simulink model "LACS"  (R2016b)
settings: Solver=VariableStepAuto  StartTime=0.0  StopTime=10  RelTol=1e-3
values from neighbouring files (symbols this model uses):
  coefficient = 0.8    [LACS.sldd]
  Detal_ref = 0.00022116955850615819 0.00022116955850615819 0.00024339323736781077 0.00026784369743330114 0.00029474273075037104 0.00032433393975435165 0.00035688482250496254 0.00039268904453642435 0.00043206891122917146 0.00047537805500027884 0.00052300435183202216 0.00057537308165349073 0.00063295034678974044 0.00069624676200566427 0.00076582142849131239 0.0008422862023284908 0.000926310265386283 0.0010186250    [LACS.sldd]    (also in path_generate.m = zeros(N,1))
  driver_decel = 4.0    [LACS.sldd]
  EgoLength = 3.048    [LACS.sldd]
  egopath = 0.0 0.25 0.5 0.75 1.0 1.25 1.5 1.7500000000000002 2.0 2.25 2.5 2.75 3.0 3.25 3.5000000000000004 3.75 4.0 4.25 4.5 4.75 5.0 5.25 5.5 5.75 6.0 6.25 6.5 6.75 7.0000000000000009 7.2499999999999991 7.5 7.75 8.0 8.25 8.5 8.75 9.0 9.25 9.5 9.75 10.0 10.25 10.5 10.75 11.0 11.25 11.5 11.75 12.0 12.25 12.5 12.75 13.0 13.25 13.5 13.750000000000002 14.000000000000002 14.250000000000002 14.499999999999998 14.7    [LACS.sldd]
  egoSpdLimit_H = 150.0    [LACS.sldd]
  egoSpdLimit_L = 10.0    [LACS.sldd]
  EgoWidth = 1.628    [LACS.sldd]
  ESA_Active = 3.0    [LACS.sldd]
  ESA_mask_1 = 31.0    [LACS.sldd]
  ESA_mask_2 = 15.0    [LACS.sldd]
  ESA_mask_3 = 255.0    [LACS.sldd]
  ESA_mask_4 = 31.0    [LACS.sldd]
  ESA_Passive = 1.0    [LACS.sldd]
  ESA_Standby = 2.0    [LACS.sldd]
  g = 9.8    [LACS.sldd]
  headwayoffset = 1.524    [LACS.sldd]
  LatAccelThershold = 0.05    [LACS.sldd]
  LatDis = 0.5    [LACS.sldd]
  LatSafetyThershold = 0.5    [LACS.sldd]
  LengthObj = 3.0    [LACS.sldd]
  ObjWidth = 2.0    [LACS.sldd]
  PB1_decel = 3.0    [LACS.sldd]
  PB2_decel = 5.0    [LACS.sldd]
  PB3_decel = 8.0    [LACS.sldd]
  Phi_dot_ref = 0.00085065224568106894 0.00085065224568106894 0.000936127966106986 0.0010301682404378703 0.0011336261186052523 0.0012474385378394444 0.001372634343205976 0.0015103430260158721 0.001661804233646022 0.0018283781058153412 0.0020115564932359636 0.0022129751145658549 0.0024344267064660809 0.0026778752189651235 0.0029454711038487576 0.0032395677369184911 0.0035627390050890382 0.0039177980756855638 0.004    [LACS.sldd]    (also in path_generate.m = zeros(N,1))
  Phi_ref = 0.00038406250525431664 0.00042271073336932769 0.00046524334565338114 0.00051204974395873044 0.000563558155980624 0.00062023946191088657 0.00068261138880285879 0.00075124310596315759 0.0008267602572639512 0.0009098504689462523 0.0010012693742370194 0.0011018471988988175 0.0012124959546271103 0.0013342172899504143 0.0014681110508986705 0.0016153846060911084 0.0017773629929370329 0.001955499943191484    [LACS.sldd]    (also in path_generate.m = phi_ref)
  SteerAngleLimit = 20.0    [LACS.sldd]
  SteerAngleSpdLimit = 20.0    [LACS.sldd]
  StrAngSpdThershold = 0.05    [LACS.sldd]
  StrAngThershold = 0.0    [LACS.sldd]
  Time2React = 1.2    [LACS.sldd]
  timeMargin = 0.5    [LACS.sldd]
  TTCthreshold1 = 2.5    [LACS.sldd]
  TTCthreshold3 = 1.0    [LACS.sldd]
  X_dot_ref = 10.0 10.0 10.0 9.9999999999999947 10.0 10.0 10.0 10.0 10.0 10.0 10.0 10.0 10.0 10.0 10.0 10.000000000000018 10.0 10.0 10.0 10.0 10.0 10.0 10.0 10.0 10.0 10.0 10.0 10.0 10.0 10.0 10.0 10.0 10.0 10.0 10.0 10.0 10.0 10.0 10.0 10.0 10.0 10.0 10.0 10.0 10.0 10.0 10.0 10.0 10.0 10.0 10.0 10.0 10.0 10.0 10.0 10.0 10.0 10.0 10.0 10.0 10.0 10.0 10.0 9.9999999999999289 10.0 10.0 10.0 10.0 10.0 10.0 10.0 10.    [LACS.sldd]    (also in path_generate.m = zeros(N,1))
  X_ref = 0.05 0.55 1.05 1.55 2.05 2.55 3.05 3.55 4.05 4.55 5.05 5.55 6.05 6.55 7.05 7.55 8.05 8.55 9.05 9.55 10.05 10.55 11.05 11.55 12.05 12.55 13.05 13.55 14.05 14.55 15.05 15.55 16.05 16.55 17.05 17.55 18.05 18.55 19.05 19.55 20.05 20.55 21.05 21.55 22.05 22.55 23.05 23.55 24.05 24.55 25.05 25.55 26.05 26.55 27.05 27.55 28.05 28.55 29.05 29.55 30.05 30.55 31.05 31.55 32.05 32.55 33.05 33.55 34.05 34.55    [LACS.sldd]    (also in path_generate.m = X_phi')
  Y_dot_ref = 0.0044363771042237217 0.0044363771042237217 0.00488273213335339 0.0053739322979981 0.0059144698111347933 0.0065092840662692251 0.0071638055584438178 0.0078840039934084845 0.0086764409570179273 0.0095483275445279979 0.01050758737719603 0.011562925461771293 0.012723903376023141 0.014001021290828194 0.015405807364013962 0.016950915064438028 0.018650229002128878 0.020518979854070446 0.0225738689793052    [LACS.sldd]    (also in path_generate.m = zeros(N,1))
  Y_ref = 0.0020016327462461514 0.0022031718511841521 0.0024249907063953382 0.0026691273130630077 0.0029378239279629127 0.0032335474185196523 0.0035590116218331136 0.0039172018997553045 0.0043114020994257287 0.0047452241472766251 0.005222640524503025 0.0057480198933628265 0.0063261661664513911 0.0069623613352525482 0.0076624123997939579 0.008432702767994656 0.0092802485212165574 0.010212759971323001 0.01123    [LACS.sldd]    (also in path_generate.m = zeros(N,1))
undefined symbols (not defined in the file or in its folder): ADR_ADRCycleTime, ADR_SteeringYawrateThresh_p, AEB_mask1, aubr, CAEB_AccelPdlPosLimit, CAEB_AccelPdlPosSpdThreshold, CAEB_CalAEBLongVelObjLimit_mps, CAEB_CalAEBVMaxDec_kmph, ESA_AESACTIVE, ESA_ERROR, ESA_ESAFunctionOFF, ESA_ESAFunctionON, ESA_ESASwichOFF, ESA_ESS_DriverSteeringNumThreshold, ESA_ESSACTIVE, ESA_ForewardCollissionLevel2, ESA_ForewardCollissionLevel3, ESA_OFF, ESA_PASSIVE, ESA_PLAN_AES, ESA_PLAN_ESSLEFT, ESA_PLAN_ESSRIGHT, ESA_PLAN_FAILURE, ESA_PLAN_OFF, ESA_PLAN_STANDBY, ESA_PLAN_WAIT, ESA_SPEEDLIMITH6_p, ESA_SPEEDLIMITH7_p, ESA_SPEEDLIMITL6_p, ESA_SPEEDLIMITL7_p, ESA_STANDBY, ESA_StrAngSpdT6_p, FromAngle2Rad, Kp, magnitude, tablebr, TTCthreshold, vubr
libraries: simulink x15, Solver_SF x9, simulink_extras x1
(part 1 of 5)
settings Model: DataDictionary=LACS.sldd  NumberOfSteps=100  Creator=NEUSOFT  LastModifiedBy=NEUSOFT

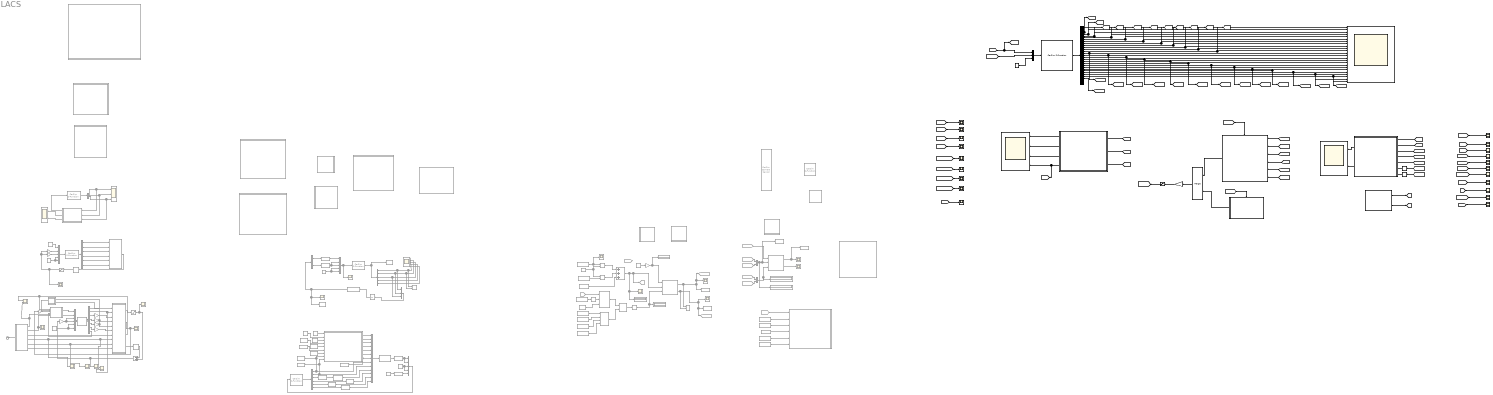
== system LACS ==
  note: 输入是制动压力
  note: 规划接口
  note: 转向不足
  note: 判断条件：
      | 1.前车静止或运动，自车与前车的关系
      | 2.TTC
      | 3.目标纵向速度
      | 4.目标纵向距离
      | 5.自车速度
      | 6.方向盘角度
      | 7.方向盘角速度
      | 8.没有刹车动作
      | 9.没有急加速动作
      | 10.航向角判断
  AEB : Subsystem  Commented=on
  AEB/ESA Comprehensive Decision : Stateflow chart  Commented=on  TreatAsAtomicUnit=on
  AEB/ESA Comprehensive Decision1 : Stateflow chart  Commented=on  TreatAsAtomicUnit=on
  AEB/ESAModeSwitch : Subsystem  Commented=on
  AEB_System : Subsystem  Commented=on
  AEBsts : Subsystem
  Add : Sum  Commented=on  Inputs=-+
  Add1 : Sum  Commented=on  Inputs=+++
  Bus Creator : BusCreator  Commented=on  Inputs=2
  Bus Creator1 : BusCreator  Commented=on  Inputs=2
  CTRL : Subsystem  Commented=on
  CarSim Camera Sensor : Solver_SF/CarSim Camera Sensor  Priority=1  Commented=on
  CarSim S-Function : Solver_SF/CarSim S-Function  Priority=1  Commented=on  SIMFILE=Simfile.sim
  CarSim S-Function1 : Solver_SF/CarSim S-Function  Priority=1  Commented=on  SIMFILE=simfile.sim
  CarSim S-Function2 : Solver_SF/CarSim S-Function  Priority=1  Commented=on  SIMFILE=simfile.sim
  CarSim S-Function2v : Solver_SF/CarSim S-Function2v  Priority=1  Commented=on  SIMFILE=[]
  CarSim S-Function3 : Solver_SF/CarSim S-Function  Priority=1  SIMFILE=simfile.sim
  CarSim S-Function4 : Solver_SF/CarSim S-Function  Priority=1  Commented=on  SIMFILE=simfile
  CarSim S-Function5 : Solver_SF/CarSim S-Function  Priority=1  Commented=on  SIMFILE=simfile.sim
  CarSim S-Function6 : Solver_SF/CarSim S-Function  Priority=1  Commented=on  SIMFILE=[]
  Clock : Clock  Commented=on
  Constant{,2,4,28} (4 alike) : Constant  Commented=on  Value=0
  Constant1 : Constant  Commented=on  Value=0.15
  Constant10 : Constant  Commented=on  Value=0.67
  Constant11 : Constant  Commented=on  Value=3
  Constant12 : Constant  Commented=on  Value=3
  Constant13 : Constant  Commented=on  Value=10
  Constant14 : Constant  Commented=on  Value=ObjWidth
  Constant15 : Constant  Commented=on  Value=10
  Constant16 : Constant  Commented=on  Value=EgoWidth
  Constant17 : Constant  Commented=on  Value=LatDis
  Constant18 : Constant  Commented=on  Value=coefficient
  Constant19 : Constant  Commented=on  Value=g
  Constant20 : Constant  Commented=on  Value=ObjWidth
  Constant21 : Constant  Commented=on  Value=X_ref
  Constant22 : Constant  Commented=on  Value=Y_ref
  Constant23 : Constant  Commented=on  Value=Phi_ref
  Constant24 : Constant  Commented=on  Value=X_dot_ref
  Constant25 : Constant  Commented=on  Value=Y_dot_ref
  Constant26 : Constant  Commented=on  Value=Phi_dot_ref
  Constant27 : Constant  Commented=on  Value=Detal_ref
  Constant29 : Constant  Commented=on  Value=10
  Constant30 : Constant  Value=0.5
  Constant5 : Constant  Commented=on  Value=1.5
  Constant6 : Constant  Commented=on  Value=0.5
  Constant7 : Constant  Commented=on  Value=2
  Constant8 : Constant  Commented=on  Value=0.8
  Constant9 : Constant  Commented=on  Value=9.8
  Delay : Delay  Commented=on  DelayLength=1  UseCircularBuffer=on
  Delay1 : Delay  DelayLength=1
  Delay2 : Delay  DelayLength=1
  Demux : Demux  Commented=on  Outputs=3
  Demux1 : Demux  Commented=on  Outputs=6
  Demux2 : Demux  Commented=on  Outputs=7
  Demux3 : Demux  Outputs=25
  Demux4 : Demux  Commented=on  Outputs=2
  Demux5 : Demux  Commented=on  Outputs=5
  Demux6 : Demux  Commented=on  Outputs=6
  Display{,1..4} (5 alike) : Display  Commented=on
  Divide : Product  Commented=on  Inputs=*/
  Divide1 : Product  Commented=on  Inputs=/*
  Divide2 : Product  Commented=on  Inputs=****
  Divide3 : Product  Commented=on  Inputs=***
  Divide4 : Product  Commented=on  Inputs=*/
  ESA : Subsystem  Commented=on
  ESAManager : Stateflow chart  Commented=on  TreatAsAtomicUnit=on
  ESARegulator_NOTON : Subsystem
  ESARegurator_ON : Subsystem
  ESAsts : Subsystem
  Fcn : Fcn  Commented=on  Expr=u*3.6
  Fcn1 : Fcn  Commented=on  Expr=u*180/pi
  Fcn2 : Fcn  Commented=on  Expr=u/180*pi
  Fcn3 : Fcn  Commented=on  Expr=u/pi*180
  Fcn4 : Fcn  Commented=on  Expr=u*3.6
  Fcn5 : Fcn  Commented=on  Expr=u/3.6
  Fcn6 : Fcn  Commented=on  Expr=u/3.6
  Fcn7 : Fcn  Commented=on  Expr=u/180*pi
  From17 : From  Commented=on  GotoTag=ye  TagVisibility=global
  From18 : From  Commented=on  GotoTag=egoSpd  TagVisibility=global
  From19 : From  Commented=on  GotoTag=egoSpd  TagVisibility=global
  From20 : From  Commented=on  GotoTag=L_prepoint  TagVisibility=global
  From21 : From  Commented=on  GotoTag=Xo  TagVisibility=global
  From22 : From  Commented=on  GotoTag=Yo  TagVisibility=global
  From23 : From  Commented=on  GotoTag=ego_path_x
  From24 : From  Commented=on  GotoTag=ego_path_y
  Gain : Gain  Commented=on  Gain=180/pi
  Gain1 : Gain  Commented=on  Gain=180/pi
  Gain2 : Gain  Commented=on  Gain=1/3.6
  Gain3 : Gain  Commented=on  Gain=1/3.6
  Gain4 : Gain  Commented=on  Gain=pi/180
  Gain5 : Gain  Commented=on  Gain=180/pi
  Gain6 : Gain  Commented=on  Gain=pi/180
  Gain7 : Gain  Commented=on  Gain=-1
  Gain8 : Gain  Gain=15.6
  Gain9 : Gain  Commented=on  Gain=1/3.6
  Goto26 : Goto  Commented=on  GotoTag=ye  TagVisibility=global
  Goto27 : Goto  Commented=on  GotoTag=ego_path_x
  Goto28 : Goto  Commented=on  GotoTag=ego_path_y
  LQR : Subsystem  Commented=on
  LatParamCaculation : Subsystem
  MATLAB Function : MATLAB Function  Commented=on  TreatAsAtomicUnit=on
  MATLAB Function1 : MATLAB Function  Commented=on  TreatAsAtomicUnit=on
  MATLAB Function2 : MATLAB Function  Commented=on  TreatAsAtomicUnit=on
  Merge : Merge
  Mux : Mux  Commented=on  Inputs=5
  Mux1 : Mux  Commented=on  Inputs=6
  Mux2 : Mux  Inputs=3
  Mux3 : Mux  Commented=on  Inputs=5
  Mux4 : Mux  Commented=on  Inputs=3
  Mux5 : Mux  Commented=on  Inputs=13
  Mux6 : Mux  Commented=on  Inputs=5
  PID Controller : simulink/Continuous/PID Controller  Commented=on  Controller=PID  TimeDomain=Continuous-time  SampleTime=-1  IntegratorMethod=Forward Euler  FilterMethod=Forward Euler  Form=Parallel  UseFilter=on  ControllerParametersSource=internal  P=0  I=0  D=0  N=100  InitialConditionSource=internal  InitialConditionForIntegrator=0  InitialConditionForFilter=0  ExternalReset=none  LimitOutput=off  UpperSaturationLimit=inf  LowerSaturationLimit=-inf  LinearizeAsGain=on  AntiWindupMode=none  Kb=1  TrackingMode=off  Kt=1  PParamMin=[]  PParamMax=[]  IParamMin=[]  IParamMax=[]  DParamMin=[]  DParamMax=[]  NParamMin=[]  NParamMax=[]  KbParamMin=[]  KbParamMax=[]  KtParamMin=[]  KtParamMax=[]  POutMin=[]  POutMax=[]  IOutMin=[]  IOutMax=[]  DOutMin=[]  DOutMax=[]  NOutMin=[]  NOutMax=[]  KbOutMin=[]  KbOutMax=[]  KtOutMin=[]  KtOutMax=[]  IntegratorOutMin=[]  IntegratorOutMax=[]  FilterOutMin=[]  FilterOutMax=[]  SumOutMin=[]  SumOutMax=[]  SumI1OutMin=[]  SumI1OutMax=[]  SumI2OutMin=[]  SumI2OutMax=[]  SumI3OutMin=[]  SumI3OutMax=[]  SumDOutMin=[]  SumDOutMax=[]  SaturationOutMin=[]  SaturationOutMax=[]  IntegratorContinuousStateAttributes=''  IntegratorStateMustResolveToSignalObject=off  IntegratorRTWStateStorageClass=Auto  FilterContinuousStateAttributes=''  FilterStateMustResolveToSignalObject=off  FilterRTWStateStorageClass=Auto  DifferentiatorICPrevScaledInput=0  DifferentiatorOutMin=[]  DifferentiatorOutMax=[]
  PassengerAEBManagement : Stateflow chart  Commented=on  TreatAsAtomicUnit=on
  Planning&Controlling : Subsystem  Commented=on
  S-Function : S-Function  Commented=on  FunctionName=MPC_Controller  SFunctionDeploymentMode=off  EnableBusSupport=off
  S-Function1 : S-Function  Commented=on  FunctionName=mpc_controller  SFunctionDeploymentMode=off  EnableBusSupport=off
  Saturation : Saturate  Commented=on  UpperLimit=1.2  LowerLimit=-1.2
  Saturation1 : Saturate  Commented=on  UpperLimit=1  LowerLimit=-1
  Saturation2 : Saturate  UpperLimit=180  LowerLimit=-180
  Scope : Scope  Commented=on  NumInputPorts=3
  Scope1 : Scope  Commented=on  NumInputPorts=2
  Scope{2,4..6,8..10,14,16..20,29..30} (15 alike) : Scope  Commented=on
  Scope11 : Scope  NumInputPorts=24
  Scope12 : Scope  NumInputPorts=4
  Scope13 : Scope  NumInputPorts=2
  Scope15 : Scope  Commented=on  NumInputPorts=5
  Scope{21..28,31..42} (20 alike) : Scope
  Scope3 : Scope  Commented=on  NumInputPorts=2
  Scope7 : Scope  Commented=on  NumInputPorts=2
  Sqrt : Sqrt  Commented=on  SaturateOnIntegerOverflow=on
  Sqrt1 : Sqrt  Commented=on  SaturateOnIntegerOverflow=on
  Subsystem : Subsystem  Commented=on
  To Workspace : ToWorkspace  Commented=on  VariableName=u  SaveFormat=Timeseries  SampleTime=-1
  To Workspace1 : ToWorkspace  Commented=on  VariableName=y  SaveFormat=Timeseries  SampleTime=-1
  To Workspace2 : ToWorkspace  Commented=on  VariableName=ego_path_y  SaveFormat=Structure With Time  SampleTime=-1
  To Workspace3 : ToWorkspace  Commented=on  VariableName=simout1  SaveFormat=Structure With Time  SampleTime=-1
  To Workspace4 : ToWorkspace  Commented=on  VariableName=ego_path_x  SaveFormat=Structure With Time  SampleTime=-1
  To Workspace5 : ToWorkspace  Commented=on  VariableName=simout2  SaveFormat=Structure With Time  SampleTime=-1
  To Workspace6 : ToWorkspace  Commented=on  VariableName=car_x  SampleTime=0.1
      settings: Save2DSignal=2-D array (concatenate along first dimension)
  To Workspace7 : ToWorkspace  Commented=on  VariableName=car_y  SampleTime=0.1
      settings: Save2DSignal=2-D array (concatenate along first dimension)
  To Workspace8 : ToWorkspace  Commented=on  VariableName=car_steer  SampleTime=0.1
      settings: Save2DSignal=2-D array (concatenate along first dimension)
  TroqueOutput : Subsystem  Commented=on
  Unit Delay : UnitDelay  Commented=on  SampleTime=-1
  XY Graph : simulink/Sinks/XY Graph  Commented=on  xmin=-1  xmax=1  ymin=-1  ymax=1  st=-1
  XY Graph1 : simulink/Sinks/XY Graph  Commented=on  xmin=-10  xmax=10  ymin=-10  ymax=10  st=-1
  double_pid_controller : Subsystem  Commented=on
  planning : MATLAB Function  Commented=on  TreatAsAtomicUnit=on
  trajectoryPlanning1 : MATLAB Function  Commented=on  TreatAsAtomicUnit=on
  trajectoryPlanning2 : MATLAB Function  Commented=on  TreatAsAtomicUnit=on
  trajectoryPlanning3 : MATLAB Function  Commented=on  TreatAsAtomicUnit=on
  trajectoryPlanning4 : MATLAB Function  Commented=on  TreatAsAtomicUnit=on
  trajectoryPlanning5 : MATLAB Function  Commented=on  TreatAsAtomicUnit=on
  trajectoryPlanning6 : MATLAB Function  Commented=on  TreatAsAtomicUnit=on
  tag scope: Angle_C2C=global, Angle_C2L=global, Angle_C2R=global, Angle_ego2obj=global, Dis_rel=global, ID_Obj=global, L_prepoint=global, L_x=global, LatAcc=global, LongiAcc=global, Mng_Obj=global, Spd_rel=global, SteerAngSpd=global, SteerAngle=global, Warning_L=global, Warning_R=global, Width_Obj=global, Xo=global, Xo_Obj=global, Yaw=global, YawRate=global, Yo=global, Yo_Obj=global, egoSpd=global, egospd_y=global
  wires:
  AEB_System/1(CMpa) -> CarSim S-Function/1
  CarSim S-Function/1 -> Demux/1
  Demux/1 -> AEB_System/1(Distance), Scope/1
  Demux/2 -> Scope/2, AEB_System/2(V_difference)
  Demux/3 -> AEB_System/3("V_Speed "), Scope/3
  AEB_System/2("Alart ") -> Scope1/1
  AEB_System/3("Break_signal ") -> Scope1/2
  CarSim S-Function1/1 -> Demux1/1
  Mux/1 -> CarSim S-Function1/1
  Demux1/1 -> Subsystem/1(x)  "x"
  Demux1/2 -> Subsystem/2(y)  "y"
  Demux1/3 -> Subsystem/3(phi)  "phi"
  Demux1/4 -> Subsystem/4(vx)  "vx"
  Demux1/5 -> Subsystem/5(vy)  "vy"
  Demux1/6 -> Subsystem/6(phi_dot)  "phi_dot"
  Subsystem/1(angle) -> Delay/1
  Gain/1 -> Mux/2
  Gain1/1 -> Mux/3
  Delay/1 -> Saturation/1
  Constant/1 -> Mux/4, Mux/5
  Constant1/1 -> Mux/1
  Saturation/1 -> Scope2/1, Gain1/1, Gain/1
  CarSim S-Function2/1 -> Demux2/1
  Mux1/1 -> CarSim S-Function2/1
  Demux2/1 -> LQR/1(x)  "x"
  Demux2/2 -> Scope3/2, LQR/2(y)  "y"
  Demux2/3 -> Gain4/1  "yaw"
  Demux2/4 -> Gain2/1  "vx"
  Demux2/5 -> Gain3/1  "vy"
  Demux2/6 -> Gain6/1  "dyaw"
  Gain3/1 -> MATLAB Function/2(vy), LQR/5(vy)
  Gain4/1 -> LQR/3(phi)
  Gain6/1 -> LQR/6(phi_dot)
  Demux2/7 -> double_pid_controller/4(rpm)  "rpm"
  double_pid_controller/1(Out1) -> Mux1/1
  double_pid_controller/2(Out2) -> Mux1/2
  Gain2/1 -> MATLAB Function/1(vx), LQR/4(vx)
  MATLAB Function/1(v) -> double_pid_controller/2(v)
  Clock/1 -> planning/1(t)
  planning/1(vp) -> Scope7/2, double_pid_controller/5(vp)  "vp"
  planning/2(ap) -> Scope6/1, double_pid_controller/6(ap)  "ap"
  planning/3(xr) -> LQR/7(xr)
  planning/4(yr) -> Scope8/1, Scope3/1, LQR/8(yr)
  planning/5(thetar) -> Scope9/1, LQR/9(thetar)
  LQR/3(s_dot) -> double_pid_controller/1(s_dot), Scope7/1
  LQR/2(es) -> Scope5/1, Gain7/1
  LQR/1(angle) -> Saturation1/1
  Constant2/1 -> Mux1/5, Mux1/6
  Gain7/1 -> double_pid_controller/3(es)
  LQR/4(ed) -> PID Controller/1
  PID Controller/1 -> Add/1
  Saturation1/1 -> Scope4/1, Add/2
  Add/1 -> Scope10/1, Gain5/1
  Gain5/1 -> Mux1/4, Mux1/3
  planning/6(kr) -> LQR/10(kappar)
  Mux2/1 -> CarSim S-Function3/1
  AEBsts/4(decel) -> [CMpa], Scope12/4
  AEBsts/3(AEBsts) -> Scope12/3
  AEBsts/2(FCW_Active) -> Scope12/2
  AEBsts/1(collision) -> Scope12/1
  CarSim S-Function3/1 -> Demux3/1
  Demux3/23 -> [Yo_Obj], Scope11/23  "目标物的横坐标"
  Demux3/22 -> [Xo_Obj], Scope11/22  "目标物的纵坐标"
  Demux3/20 -> [L_prepoint], Scope11/20  "纵向预瞄点"
  Demux3/24 -> [SteerAngSpd], Scope11/24  "方向盘角速度"
  Demux3/21 -> [L_x], Scope11/21  "纵坐标"
  Demux3/19 -> [Yo], Scope11/19  "车辆质心的全局Y坐标"
  Demux3/18 -> [Xo], Scope11/18  "车辆质心的全局X坐标"
  Demux3/17 -> [YawRate], Scope11/17  "车辆航向角的导数"
  Demux3/16 -> [LatAcc], Scope11/16  "横向加速度"
  Demux3/15 -> [LongiAcc], Scope11/15  "纵向加速度"
  Demux3/14 -> [Yaw], Scope11/14  "航向角"
  Demux3/13 -> [SteerAngle], Scope11/13  "方向盘转角"
  Demux3/12 -> [Angle_ego2obj], Scope11/12  "本车与物体垂向的方位角"
  Demux3/11 -> [Angle_C2R], Scope11/11  "相对传感器瞄准的方向，到物体最右侧直线的方位角"
  Demux3/10 -> [Angle_C2L], Scope11/10  "相对传感器瞄准的方向，到物体最左侧直线的方位角"
  Demux3/9 -> [Angle_C2C], Scope11/9  "相对传感器瞄准的方向，到物体最近点直线的方位角"
  Demux3/8 -> [Warning_R], Scope11/8  "右侧预警"
  Demux3/7 -> [Warning_L], Scope11/7  "左侧预警"
  Demux3/6 -> [Mng_Obj], Scope11/6  "置信度"
  Demux3/5 -> [Width_Obj], Scope11/5  "目标宽度"
  Demux3/4 -> [ID_Obj], Scope11/4  "目标ID"
  Demux3/3 -> Scope11/3, [egoSpd]  "纵向速度"
  Demux3/2 -> Scope11/2, [Spd_rel]  "相对速度"
  Demux3/1 -> [Dis_rel], Scope11/1  "相对距离"
  [ESA_Active] -> ESARegurator_ON/Action
  [ESA_NOTActive] -> ESARegulator_NOTON/Action
  ESARegurator_ON/1(WheelSteerAngle) -> Merge/1
  ESARegulator_NOTON/1(WheelSteerAngle) -> Merge/2
  ESAsts/2(ESAsts) -> Scope13/2
  Merge/1 -> Gain8/1
  [Dis_rel] -> AEBsts/1(LongiDis)
  [Spd_rel] -> AEBsts/2(LongiVel)
  [egoSpd] -> AEBsts/3(EgoSpd)
  [Dis_rel] -> ESAsts/1(LongiDis)
  [Spd_rel] -> ESAsts/2(LongiVel)
  [SteerAngSpd] -> ESAsts/4(SteerAngleSpd)
  [SteerAngle] -> ESAsts/3(SteerAngle)
  [LatAcc] -> ESAsts/5(LatAccel)
  Mux3/1 -> Scope16/1, CarSim S-Function4/1
  Fcn/1 -> Mux3/1  "Speed"
  Fcn1/1 -> Mux3/3, Mux3/2  "Steer_R1"
  Constant4/1 -> Mux3/5, Mux3/4  "Steer_R2"
  Demux4/1 -> Fcn/1  "V"
  Demux4/2 -> Fcn1/1  "δ"
  S-Function/1 -> Scope14/1, To Workspace/1, Demux4/1
  Unit Delay/1 -> S-Function/1
  CarSim S-Function4/1 -> Demux5/1, To Workspace1/1
  Demux5/1 -> Mux4/1, XY Graph/1, Scope15/1  "X0"
  Demux5/2 -> Mux4/2, XY Graph/2, Scope15/2  "Y0"
  Demux5/3 -> Mux4/3, Scope15/3  "Yaw"
  Demux5/4 -> Scope15/4  "Vx"
  Demux5/5 -> Scope15/5  "Steer_SW"
  Mux4/1 -> Unit Delay/1
  [CMpa] -> [CMpa_M], Mux2/1
  [SteerAngle_Out] -> Mux2/2
  Constant14/1 -> Scope29/1, Divide/1
  Constant7/1 -> Divide/2, Divide1/1
  Constant5/1 -> Divide1/2
  Divide1/1 -> Add1/2
  Divide/1 -> Add1/1
  Constant6/1 -> Add1/3
  Add1/1 -> Display4/1, Scope30/1, trajectoryPlanning2/2(ye), Goto26/1
  Constant11/1 -> Divide2/4
  Constant10/1 -> Divide2/3
  Constant9/1 -> Divide2/2
  Constant8/1 -> Divide2/1
  From17/1 -> Divide3/1
  Sqrt/1 -> Divide3/2
  Constant12/1 -> Sqrt/1
  Constant13/1 -> Divide3/3
  Divide3/1 -> Divide4/1
  Divide2/1 -> Divide4/2
  Divide4/1 -> Sqrt1/1
  Sqrt1/1 -> trajectoryPlanning2/3(te), Display/1
  Gain9/1 -> trajectoryPlanning2/1(v_x), Display1/1
  trajectoryPlanning2/1(egopath_x) -> XY Graph1/1, Goto27/1, Scope18/1, To Workspace4/1
  trajectoryPlanning2/2(egopath_y) -> XY Graph1/2, Scope17/1, Goto28/1, To Workspace2/1
  From20/1 -> trajectoryPlanning3/1(ld_veh)
  From21/1 -> Bus Creator/1
  From22/1 -> Bus Creator/2
  Bus Creator/1 -> Display2/1, trajectoryPlanning3/3("currentPose ")
  From23/1 -> Bus Creator1/1
  From24/1 -> Bus Creator1/2
  trajectoryPlanning3/1(ld_pre) -> To Workspace5/1, Scope19/1
  Bus Creator1/1 -> Display3/1, trajectoryPlanning3/2(refpath), To Workspace3/1
  trajectoryPlanning3/2(currentPose) -> Scope20/1
  [te] -> Delay2/1
  [ye] -> Delay1/1
  Delay2/1 -> ESAsts/7(te)
  [TTC_M] -> Scope23/1
  [CMpa_M] -> Scope21/1
  [Longivel_M] -> Scope24/1
  [LongiDis_M] -> Scope25/1
  [FCWStopTime_M] -> Scope22/1
  [PB1StoppingTime_M] -> Scope26/1
  [PB2StoppingTime_M] -> Scope27/1
  [FBStoppingTime] -> Scope28/1
  [ESA_sts_M] -> Scope31/1
  [Dis_rel] -> Scope32/1
  [Spd_rel] -> Scope33/1
  [SteerAngle] -> Scope34/1
  [SteerAngle_Out] -> Scope37/1
  [LatAcc] -> Scope36/1
  [SteerAngSpd] -> Scope35/1
  [LatDisLimit_c] -> Scope40/1
  [TTC] -> Scope39/1
  [Allow2Str] -> Scope38/1
  ESAsts/1(collision) -> Scope13/1
  Delay1/1 -> ESAsts/6(ye)
  Gain8/1 -> Saturation2/1
  Saturation2/1 -> [SteerAngle_Out]
  Constant15/1 -> Gain9/1
  Constant19/1 -> trajectoryPlanning6/6(g)
  Constant18/1 -> trajectoryPlanning6/5(coefficient)
  Constant17/1 -> trajectoryPlanning6/4(EgoWidth)
  Constant16/1 -> trajectoryPlanning6/3(ObjWidth)
  Constant20/1 -> trajectoryPlanning6/2(LatDis)
  From18/1 -> trajectoryPlanning6/1(v_x)
  Constant21/1 -> MATLAB Function1/1(X_ref)
  Constant22/1 -> MATLAB Function1/2(Y_ref)
  Constant23/1 -> MATLAB Function1/3(Phi_ref)
  Constant24/1 -> MATLAB Function1/4(X_dot_ref)
  Constant25/1 -> MATLAB Function1/5(Y_dot_ref)
  Constant26/1 -> MATLAB Function1/6(Phi_dot_ref)
  Constant27/1 -> MATLAB Function1/7(Detal_ref)
  MATLAB Function1/5(y_dot_ref) -> Mux5/5
  MATLAB Function1/1(x_ref) -> Mux5/1
  MATLAB Function1/2(y_ref) -> Mux5/2
  MATLAB Function1/3(phi_ref) -> Mux5/3
  MATLAB Function1/4(x_dot_ref) -> Mux5/4
  MATLAB Function1/6(phi_dot_ref) -> Mux5/6
  MATLAB Function1/7(detal_ref) -> To Workspace8/1, Mux5/7
  Mux5/1 -> S-Function1/1
  CarSim S-Function5/1 -> Demux6/1
  Demux6/1 -> MATLAB Function1/8(x), To Workspace6/1, Mux5/8
  Demux6/2 -> MATLAB Function1/9(y), To Workspace7/1, Mux5/9
  Demux6/4 -> Fcn5/1
  Demux6/5 -> Fcn6/1
  Demux6/6 -> Fcn7/1
  Demux6/3 -> Fcn2/1
  Fcn2/1 -> MATLAB Function2/1(u)
  MATLAB Function2/1(yaw) -> Mux5/10
  Constant28/1 -> Mux6/3, Mux6/4
  Fcn3/1 -> Mux6/1, Mux6/2
  S-Function1/1 -> Fcn3/1
  Constant29/1 -> Fcn4/1
  Fcn4/1 -> Mux6/5
  Mux6/1 -> CarSim S-Function5/1
  Fcn5/1 -> Mux5/11
  Fcn6/1 -> Mux5/12
  Fcn7/1 -> Mux5/13
  Constant30/1 -> Mux2/3
  LatParamCaculation/2(te) -> [te]
  LatParamCaculation/1(ye) -> [ye]
  [Xo] -> ESARegurator_ON/1(Xo)
  [Yo] -> ESARegurator_ON/2(Yo)
  [Yaw] -> ESARegurator_ON/3(Yaw)
  [YawRate] -> ESARegurator_ON/6(YawRate)
  Demux3/25 -> [egospd_y]
  [egoSpd] -> ESARegurator_ON/4(X_dot)
  [egospd_y] -> ESARegurator_ON/5(Y_dot)
  [egoSpd] -> Scope41/1
  [egoSpd] -> Scope42/1

== system LACS/AEB ==
  LongiVel : Inport
  LongiDis : Inport  Port=2
  ConditionAdaptAEB : Subsystem
  DrvRapidAccelAction : Subsystem  Commented=on
  TTCCaculation : Subsystem
  Out1 : Outport
  Out3 : Outport  Port=2
  Out4 : Outport  Port=3
  Out5 : Outport  Port=4
  Out6 : Outport  Port=5
  Out7 : Outport  Port=6
  Out8 : Outport  Port=7
  Out10 : Outport  Port=8
  wires:
  ConditionAdaptAEB/6(Out6) -> Out7/1
  ConditionAdaptAEB/5(Out5) -> Out6/1
  ConditionAdaptAEB/2(Out2) -> Out3/1
  ConditionAdaptAEB/8(Out8) -> Out10/1
  ConditionAdaptAEB/7(Out7) -> Out8/1
  ConditionAdaptAEB/3(Out3) -> Out4/1
  ConditionAdaptAEB/1(Out1) -> Out1/1
  ConditionAdaptAEB/4(Out4) -> Out5/1
  LongiVel/1 -> TTCCaculation/1(LongiVel)
  LongiDis/1 -> TTCCaculation/2(LongiDis)

== system LACS/AEB//ESAModeSwitch ==
  SteerAngle : Inport
  SteerAngleSpd : Inport  Port=2
  AEBTTC : Inport  Port=3
  EgoSpd : Inport  Port=4
  If : If  IfExpression=u1==1
  If Action Subsystem : Subsystem  TreatAsAtomicUnit=on
  If Action Subsystem1 : Subsystem  TreatAsAtomicUnit=on
  Merge : Merge
  Merge1 : Merge
  Relational Operator22 : RelationalOperator  Operator=<=  OutDataTypeStr=boolean  RndMeth=Simplest
  Subsystem : Subsystem
  TTC1 : Constant  Value=6  OutDataTypeStr=boolean
  ESATakeOverReq : Outport
  AEBCrashAvoid : Outport  Port=2
  wires:
  If/1 -> If Action Subsystem/Action
  If/2 -> If Action Subsystem1/Action
  SteerAngle/1 -> Subsystem/1(SteerAngle)
  SteerAngleSpd/1 -> Subsystem/2(SteerAngleSpd)
  Subsystem/1(DrvRapidSteerAction) -> If/1
  EgoSpd/1 -> If Action Subsystem1/2(EgoSpd)
  AEBTTC/1 -> If Action Subsystem1/3(AEBTTC), Relational Operator22/1
  TTC1/1 -> Relational Operator22/2
  Relational Operator22/1 -> If Action Subsystem1/1(AEBTTCVaild)
  Merge/1 -> ESATakeOverReq/1
  Merge1/1 -> AEBCrashAvoid/1
  If Action Subsystem/1(ESAVTakeOverReq) -> Merge/1
  If Action Subsystem1/1(ESAVTakeOverReq) -> Merge/2
  If Action Subsystem/2(AEBVCrashAvoid) -> Merge1/1
  If Action Subsystem1/2(AEBVCrashAvoid) -> Merge1/2

== system LACS/AEB_System ==
  Distance : Inport
  V_difference : Inport  Port=2
  "V_Speed " : Inport  Port=3
  Chart : Stateflow chart  TreatAsAtomicUnit=on
  CMpa : Outport
  "Alart " : Outport  Port=2
  "Break_signal " : Outport  Port=3
  wires:
  Distance/1 -> Chart/1(Distance)
  V_difference/1 -> Chart/2(V_difference)
  "V_Speed "/1 -> Chart/3(V_Speed)
  Chart/1(CMpa) -> CMpa/1
  Chart/2(Alart) -> "Alart "/1
  Chart/3(Break_signal) -> "Break_signal "/1

== system LACS/AEBsts ==
  LongiDis : Inport
  LongiVel : Inport  Port=2
  EgoSpd : Inport  Port=3
  AEB_sts : Stateflow chart  TreatAsAtomicUnit=on
  Brake2StopTime : Subsystem
  Constant1 : Constant  Value=PB2_decel
  Constant2 : Constant  Value=PB3_decel
  Constant3 : Constant  Value=PB1_decel
  Constant6 : Constant  Value=0.1
  Relational Operator4 : RelationalOperator  Operator=<  OutDataTypeStr=boolean  RndMeth=Simplest
  TTCCaculation : Subsystem
  collision : Outport
  FCW_Active : Outport  Port=2
  AEBsts : Outport  Port=3
  decel : Outport  Port=4
  wires:
  TTCCaculation/1(collision) -> collision/1
  EgoSpd/1 -> Relational Operator4/1, Brake2StopTime/1(EgoSpd)
  Constant3/1 -> AEB_sts/6(CMpa1), Brake2StopTime/2(CMpa1)
  Constant1/1 -> AEB_sts/7(CMpa2), Brake2StopTime/3(CMpa2)
  Brake2StopTime/2(PB1StoppingTime) -> AEB_sts/3(PB1time)
  Relational Operator4/1 -> AEB_sts/9(stop)
  Constant2/1 -> AEB_sts/8(CMpa3), Brake2StopTime/4(CMpa3)
  TTCCaculation/2(TTC) -> AEB_sts/1(TTC)
  LongiDis/1 -> TTCCaculation/1(LongiDis)
  LongiVel/1 -> TTCCaculation/2(LongiVel)
  Brake2StopTime/3(PB2StoppingTime) -> AEB_sts/4(PB2time)
  Constant6/1 -> Relational Operator4/2
  Brake2StopTime/4(FBStoppingTime) -> AEB_sts/5(FBtime)
  AEB_sts/2(AEBsts) -> AEBsts/1
  AEB_sts/3(decel) -> decel/1
  AEB_sts/1(FCW_Active) -> FCW_Active/1
  Brake2StopTime/1(FCWStoppingTime) -> AEB_sts/2(FCWtime)

== system LACS/CTRL ==
  planning1 : MATLAB Function  TreatAsAtomicUnit=on

== system LACS/ESA ==
  ConditionAdaptESA : Subsystem
  Control : Subsystem
  OverlapCaculation : Subsystem
  SteerDirection : Subsystem
  TrajactoryPlan : Subsystem
  wires:
  Control/1(Out1) -> ?
  TrajactoryPlan/1(Pos_ego) -> ?

== system LACS/ESARegulator_NOTON ==
  Action Port : ActionPort  ActionType=else
  Constant : Constant  Value=0
  WheelSteerAngle : Outport
  wires:
  Constant/1 -> WheelSteerAngle/1

== system LACS/ESARegurator_ON ==
  Xo : Inport
  Yo : Inport  Port=2
  Yaw : Inport  Port=3
  X_dot : Inport  Port=4
  Y_dot : Inport  Port=5
  YawRate : Inport  Port=6
  Action Port : ActionPort  ActionType=then
  Constant : Constant  Value=X_ref
  Constant1 : Constant  Value=Y_ref
  Constant2 : Constant  Value=Phi_ref
  Constant3 : Constant  Value=X_dot_ref
  Constant4 : Constant  Value=Y_dot_ref
  Constant5 : Constant  Value=Phi_dot_ref
  Constant6 : Constant  Value=Detal_ref
  Fcn : Fcn  Expr=u/180*pi
  Fcn1 : Fcn  Expr=u/pi*180
  Fcn3 : Fcn  Expr=u/3.6
  Fcn4 : Fcn  Expr=u/3.6
  Fcn5 : Fcn  Expr=u/180*pi
  MATLAB Function : MATLAB Function  TreatAsAtomicUnit=on
  MATLAB Function1 : MATLAB Function  TreatAsAtomicUnit=on
  Mux : Mux  Inputs=13
  S-Function : S-Function  FunctionName=mpc_controller  SFunctionDeploymentMode=off  EnableBusSupport=off
  To Workspace : ToWorkspace  VariableName=car_x1  SampleTime=0.0005
      settings: Save2DSignal=2-D array (concatenate along first dimension)
  To Workspace1 : ToWorkspace  VariableName=car_y1  SampleTime=0.0005
      settings: Save2DSignal=2-D array (concatenate along first dimension)
  To Workspace2 : ToWorkspace  VariableName=car_steer1  SampleTime=0.0005
      settings: Save2DSignal=2-D array (concatenate along first dimension)
  WheelSteerAngle : Outport
  wires:
  Constant/1 -> MATLAB Function/1(X_ref)
  Constant1/1 -> MATLAB Function/2(Y_ref)
  Constant2/1 -> MATLAB Function/3(Phi_ref)
  Constant3/1 -> MATLAB Function/4(X_dot_ref)
  Constant4/1 -> MATLAB Function/5(Y_dot_ref)
  Constant5/1 -> MATLAB Function/6(Phi_dot_ref)
  Constant6/1 -> MATLAB Function/7(Detal_ref)
  MATLAB Function/5(y_dot_ref) -> Mux/5
  MATLAB Function/1(x_ref) -> Mux/1
  MATLAB Function/2(y_ref) -> Mux/2
  MATLAB Function/3(phi_ref) -> Mux/3
  MATLAB Function/4(x_dot_ref) -> Mux/4
  MATLAB Function/6(phi_dot_ref) -> Mux/6
  MATLAB Function/7(detal_ref) -> Mux/7, To Workspace2/1
  Xo/1 -> Mux/8, MATLAB Function/8(x), To Workspace/1
  Yo/1 -> Mux/9, MATLAB Function/9(y), To Workspace1/1
  Mux/1 -> S-Function/1
  Fcn1/1 -> WheelSteerAngle/1
  S-Function/1 -> Fcn1/1
  Fcn/1 -> MATLAB Function1/1(u)
  Fcn5/1 -> Mux/13
  Yaw/1 -> Fcn/1
  YawRate/1 -> Fcn5/1
  Y_dot/1 -> Fcn4/1
  X_dot/1 -> Fcn3/1
  MATLAB Function1/1(yaw) -> Mux/10
  Fcn3/1 -> Mux/11
  Fcn4/1 -> Mux/12

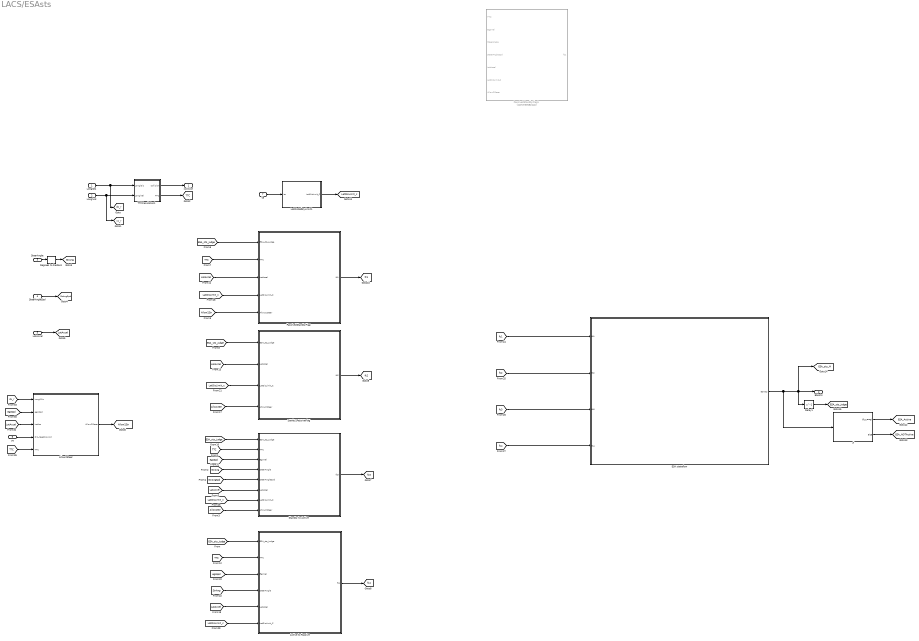
== system LACS/ESAsts ==
  LongiDis : Inport
  LongiVel : Inport  Port=2
  SteerAngle : Inport  Port=3
  SteerAngleSpd : Inport  Port=4
  LatAccel : Inport  Port=5
  ye : Inport  Port=6
  te : Inport  Port=7
  Active to Passive : Subsystem
  Allow2Steer : Subsystem
  Degrees to Radians : simulink_extras/Transformations/Degrees to Radians
  Delay1 : Delay  DelayLength=1
  ESA stateflow : Stateflow chart  TreatAsAtomicUnit=on
  If : If  IfExpression=u1==3
  LatDisSafetyLimit1 : Subsystem
  Passive2StandbyFlag : Subsystem
  Passive2StandbyFlag1 : Subsystem  Commented=on
  Stanby2PassiveFlag : Subsystem
  Standby to Active : Subsystem
  TTCCaculation1 : Subsystem
  collision : Outport
  ESAsts : Outport  Port=2
  tag scope: Allow2Str=global, ESA_Active=global, ESA_NOTActive=global, ESA_sts_Judge=global, ESA_sts_M=global, LatAccel=global, LatDisLimit_c=global, StrAng=global, StrAngSpd=global, TTC=global, dx_r=global, fc1=global, fc2=global, fc3=global, fc4=global, vx_r=global
  wires:
  LongiDis/1 -> [dx_r], TTCCaculation1/1(LongiDis)
  LongiVel/1 -> [vx_r], TTCCaculation1/2(LongiVel)
  TTCCaculation1/1(collision) -> collision/1
  [egoSpd] -> Standby to Active/3(EgoVel)
  TTCCaculation1/2(TTC) -> [TTC]
  [TTC] -> Standby to Active/2(TTC)
  [StrAng] -> Standby to Active/4(SteerAngle)
  SteerAngleSpd/1 -> [StrAngSpd]
  LatAccel/1 -> [LatAccel]
  [Allow2Str] -> Standby to Active/8(Allow2Steer)
  [StrAngSpd] -> Standby to Active/5(SteerAngleSpd)
  [LatAccel] -> Standby to Active/6(LatAccel)
  [TTC] -> Passive2StandbyFlag/2(TTC)
  Standby to Active/1(fc3) -> [fc3]
  Active to Passive/1(fc4) -> [fc4]
  Stanby2PassiveFlag/1(fc2) -> [fc2]
  Passive2StandbyFlag/1(fc1) -> [fc1]
  [fc1] -> ESA stateflow/1(fc1)
  [fc2] -> ESA stateflow/2(fc2)
  [fc3] -> ESA stateflow/3(fc3)
  [fc4] -> ESA stateflow/4(fc4)
  [Allow2Str] -> Passive2StandbyFlag/5(Allow2Steer)
  [LatAccel] -> Passive2StandbyFlag/3(LatAccel)
  LatDisSafetyLimit1/1(LatDisLimit_C) -> [LatDisLimit_c]
  [LatDisLimit_c] -> Passive2StandbyFlag/4(LatDisLimit_C)
  [LatDisLimit_c] -> Standby to Active/7(LatDisLimit_C)
  If/1 -> [ESA_Active]
  If/2 -> [ESA_NOTActive]
  Allow2Steer/1(Allow2Steer) -> [Allow2Str]
  SteerAngle/1 -> Degrees to Radians/1
  Degrees to Radians/1 -> [StrAng]
  te/1 -> LatDisSafetyLimit1/1(te)
  [TTC] -> Allow2Steer/5(TTC)
  ye/1 -> Allow2Steer/4(Dis_Need2Avoid)
  [egoSpd] -> Allow2Steer/2(egoSpd)
  [LatAccel] -> Allow2Steer/3(LatAcc)
  [dx_r] -> Allow2Steer/1(LongiDis)
  [ESA_sts_Judge] -> Passive2StandbyFlag/1(ESA_sts_Judge)
  [Allow2Str] -> Stanby2PassiveFlag/4(Allow2Steer)
  [LatDisLimit_c] -> Stanby2PassiveFlag/3(LatDisLimit_C)
  [LatAccel] -> Stanby2PassiveFlag/2(LatAccel)
  [ESA_sts_Judge] -> Stanby2PassiveFlag/1(ESA_sts_Judge)
  [ESA_sts_Judge] -> Standby to Active/1(ESA_sts_Judge)
  [LatDisLimit_c] -> Active to Passive/6(LatDisLimit_C)
  [LatAccel] -> Active to Passive/5(LatAccel)
  [StrAng] -> Active to Passive/4(SteerAngle)
  [egoSpd] -> Active to Passive/3(EgoVel)
  [TTC] -> Active to Passive/2(TTC)
  [ESA_sts_Judge] -> Active to Passive/1(ESA_sts_Judge)
  Delay1/1 -> [ESA_sts_Judge]
  ESA stateflow/1(ESAsts) -> If/1, Delay1/1, [ESA_sts_M], ESAsts/1

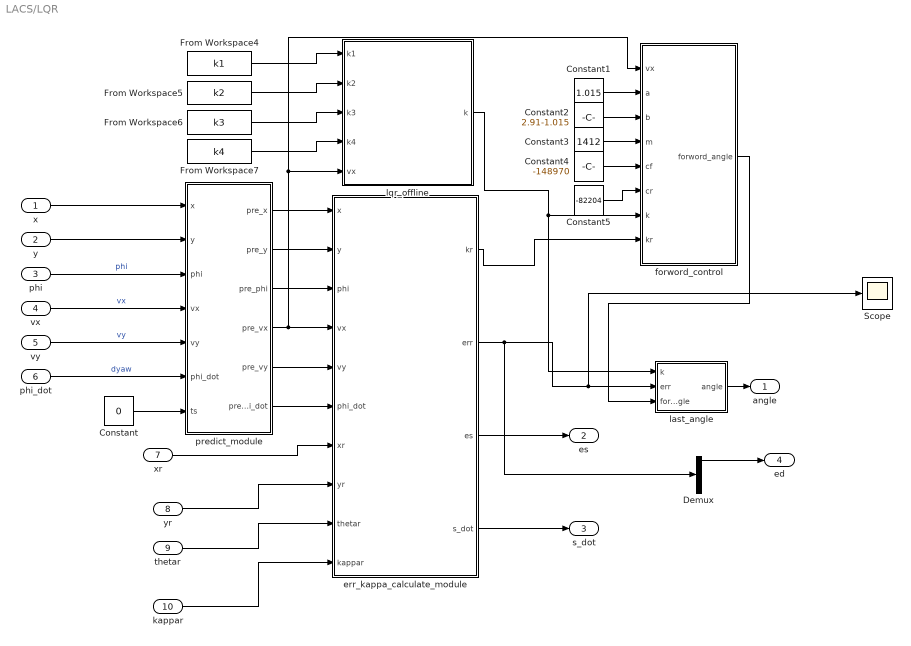
== system LACS/LQR ==
  x : Inport
  y : Inport  Port=2
  phi : Inport  Port=3
  vx : Inport  Port=4
  vy : Inport  Port=5
  phi_dot : Inport  Port=6
  xr : Inport  Port=7
  yr : Inport  Port=8
  thetar : Inport  Port=9
  kappar : Inport  Port=10
  Constant : Constant  Value=0
  Constant1 : Constant  Value=1.015
  Constant2 : Constant  Value=2.91-1.015
  Constant3 : Constant  Value=1412
  Constant4 : Constant  Value=-148970
  Constant5 : Constant  Value=-82204
  Demux : Demux
  From Workspace4 : FromWorkspace  VariableName=k1  SampleTime=0
  From Workspace5 : FromWorkspace  VariableName=k2  SampleTime=0
  From Workspace6 : FromWorkspace  VariableName=k3  SampleTime=0
  From Workspace7 : FromWorkspace  VariableName=k4  SampleTime=0
  Scope : Scope
  err_kappa_calculate_module : MATLAB Function  TreatAsAtomicUnit=on
  forword_control : MATLAB Function  TreatAsAtomicUnit=on
  last_angle : MATLAB Function  TreatAsAtomicUnit=on
  lqr_offline : MATLAB Function  TreatAsAtomicUnit=on
  predict_module : MATLAB Function  TreatAsAtomicUnit=on
  angle : Outport
  es : Outport  Port=2
  s_dot : Outport  Port=3
  ed : Outport  Port=4
  wires:
  From Workspace7/1 -> lqr_offline/4(k4)
  vy/1 -> predict_module/5(vy)  "vy"
  From Workspace6/1 -> lqr_offline/3(k3)
  x/1 -> predict_module/1(x)
  lqr_offline/1(k) -> last_angle/1(k), forword_control/7(k)
  predict_module/2(pre_y) -> err_kappa_calculate_module/2(y)
  err_kappa_calculate_module/1(kr) -> forword_control/8(kr)
  forword_control/1(forword_angle) -> last_angle/3(forword_angle)
  predict_module/4(pre_vx) -> lqr_offline/5(vx), forword_control/1(vx), err_kappa_calculate_module/4(vx)
  phi_dot/1 -> predict_module/6(phi_dot)  "dyaw"
  last_angle/1(angle) -> angle/1
  From Workspace5/1 -> lqr_offline/2(k2)
  vx/1 -> predict_module/4(vx)  "vx"
  y/1 -> predict_module/2(y)
  phi/1 -> predict_module/3(phi)  "phi"
  Constant/1 -> predict_module/7(ts)
  From Workspace4/1 -> lqr_offline/1(k1)
  predict_module/1(pre_x) -> err_kappa_calculate_module/1(x)
  predict_module/5(pre_vy) -> err_kappa_calculate_module/5(vy)
  predict_module/6(pre_phi_dot) -> err_kappa_calculate_module/6(phi_dot)
  predict_module/3(pre_phi) -> err_kappa_calculate_module/3(phi)
  Constant1/1 -> forword_control/2(a)
  Constant2/1 -> forword_control/3(b)
  Constant3/1 -> forword_control/4(m)
  Constant4/1 -> forword_control/5(cf)
  xr/1 -> err_kappa_calculate_module/7(xr)
  yr/1 -> err_kappa_calculate_module/8(yr)
  thetar/1 -> err_kappa_calculate_module/9(thetar)
  kappar/1 -> err_kappa_calculate_module/10(kappar)
  err_kappa_calculate_module/3(es) -> es/1
  err_kappa_calculate_module/4(s_dot) -> s_dot/1
  Constant5/1 -> forword_control/6(cr)
  Demux/1 -> ed/1
  err_kappa_calculate_module/2(err) -> Demux/1, Scope/1, last_angle/2(err)

== system LACS/LatParamCaculation ==
  Add : Sum  Inputs=+++
  Constant : Constant  Value=EgoWidth
  Constant1 : Constant  Value=LatDis
  Constant2 : Constant  Value=2
  Constant3 : Constant  Value=coefficient
  Constant4 : Constant  Value=g
  Constant5 : Constant  Value=0.67
  Constant6 : Constant  Value=3
  Constant7 : Constant  Value=3
  Constant8 : Constant  Value=10
  Constant9 : Constant  Value=ObjWidth
  Divide : Product  Inputs=*/
  Divide1 : Product  Inputs=/*
  Divide2 : Product  Inputs=****
  Divide3 : Product  Inputs=***
  Divide4 : Product  Inputs=*/
  Sqrt : Sqrt  SaturateOnIntegerOverflow=on
  Sqrt1 : Sqrt  SaturateOnIntegerOverflow=on
  ye : Outport
  te : Outport  Port=2
  wires:
  Constant9/1 -> Divide/1
  Constant2/1 -> Divide/2, Divide1/1
  Constant/1 -> Divide1/2
  Divide1/1 -> Add/2
  Divide/1 -> Add/1
  Constant1/1 -> Add/3
  Constant6/1 -> Divide2/4
  Constant5/1 -> Divide2/3
  Constant4/1 -> Divide2/2
  Constant3/1 -> Divide2/1
  Add/1 -> Divide3/1, ye/1
  Sqrt/1 -> Divide3/2
  Constant7/1 -> Sqrt/1
  Constant8/1 -> Divide3/3
  Divide3/1 -> Divide4/1
  Divide2/1 -> Divide4/2
  Divide4/1 -> Sqrt1/1
  Sqrt1/1 -> te/1

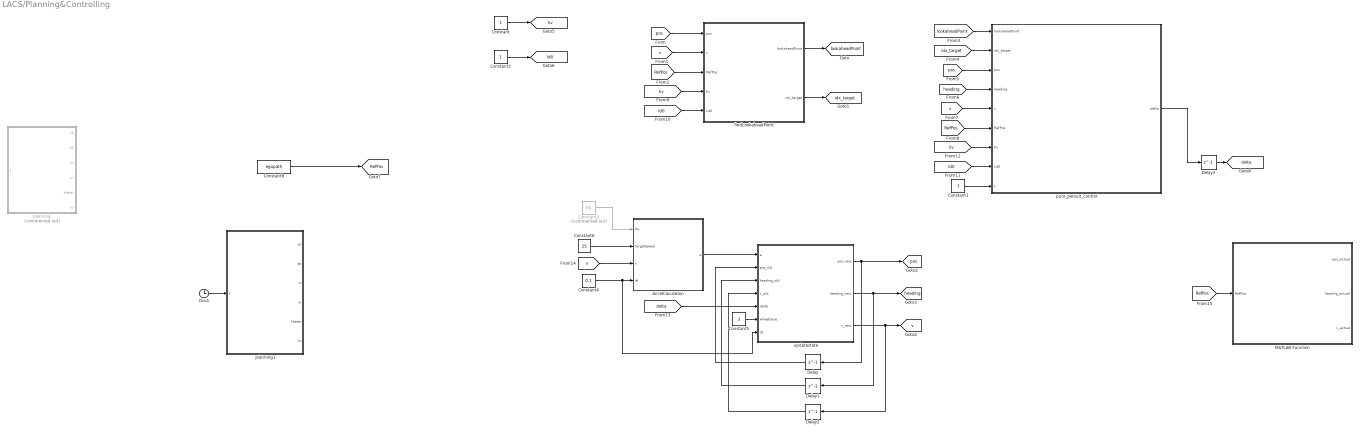
== system LACS/Planning&Controlling ==
  AccelCaculation : MATLAB Function  TreatAsAtomicUnit=on
  Clock : Clock
  Constant : Constant
  Constant1 : Constant  Value=3
  Constant2 : Constant
  Constant3 : Constant  Commented=on  Value=Kp
  Constant4 : Constant  Value=0.1
  Constant5 : Constant  Value=3
  Constant6 : Constant  Value=25
  Constant8 : Constant  Value=egopath
  Delay{,1..3} (4 alike) : Delay  DelayLength=1
  MATLAB Function : MATLAB Function  TreatAsAtomicUnit=on
  findLookaheadPoint : MATLAB Function  TreatAsAtomicUnit=on
  planning : MATLAB Function  Commented=on  TreatAsAtomicUnit=on
  planning1 : MATLAB Function  TreatAsAtomicUnit=on
  pure_persuit_control : MATLAB Function  TreatAsAtomicUnit=on
  updatestate : MATLAB Function  TreatAsAtomicUnit=on
  tag scope: RefPos=global, delta=global, heading=global, idx_target=global, kv=global, ld0=global, lookaheadPoint=global, pos=global, v=global
  wires:
  findLookaheadPoint/1(lookaheadPoint) -> [lookaheadPoint]
  findLookaheadPoint/2(idx_target) -> [idx_target]
  [pos] -> findLookaheadPoint/1(pos)
  [v] -> findLookaheadPoint/2(v)
  [RefPos] -> findLookaheadPoint/3(RefPos)
  [lookaheadPoint] -> pure_persuit_control/1(lookaheadPoint)
  [idx_target] -> pure_persuit_control/2(idx_target)
  updatestate/1(pos_new) -> Delay/1, [pos]
  [pos] -> pure_persuit_control/3(pos)
  updatestate/2(heading_new) -> Delay1/1, [heading]
  [heading] -> pure_persuit_control/4(heading)
  updatestate/3(v_new) -> Delay2/1, [v]
  [v] -> pure_persuit_control/5(v)
  [RefPos] -> pure_persuit_control/6(RefPos)
  pure_persuit_control/1(delta) -> Delay3/1
  Constant1/1 -> pure_persuit_control/9(L)
  Constant/1 -> [kv]
  Constant2/1 -> [ld0]
  [kv] -> findLookaheadPoint/4(Kv)
  [ld0] -> findLookaheadPoint/5(Ld0)
  [kv] -> pure_persuit_control/7(Kv)
  [ld0] -> pure_persuit_control/8(Ld0)
  Delay/1 -> updatestate/2(pos_old)
  Delay1/1 -> updatestate/3(heading_old)
  Delay2/1 -> updatestate/4(v_old)
  Delay3/1 -> [delta]
  [delta] -> updatestate/5(delta)
  Constant5/1 -> updatestate/6(wheelbase)
  AccelCaculation/1(a) -> updatestate/1(a)
  Constant4/1 -> updatestate/7(dt), AccelCaculation/4(dt)
  [v] -> AccelCaculation/3(v)
  Constant3/1 -> AccelCaculation/1(Kp)
  Constant6/1 -> AccelCaculation/2(targetSpeed)
  Constant8/1 -> [RefPos]
  Clock/1 -> planning1/1(t)
  [RefPos] -> MATLAB Function/1(RefPos)
